simulink model "Nexonar_Test2"  (R2018b)
settings: Solver=FixedStepDiscrete  StartTime=0.0  StopTime=10  RelTol=1e-3  EnableMultiTasking=on
settings Model: ExtModeTrigDuration=8  Creator=User  LastModifiedBy=hengw
settings DataIOCC: LimitDataPoints=on  SaveFormat=Array  SaveOutput=off  SaveTime=off
settings OptimizationCC: DefaultUnderspecifiedDataType=single  ExpressionDepthLimit=2147483647  LifeSpan=1  MaxStackSize=512
settings DebuggingCC: UnderspecifiedInitializationDetection=Classic  MergeDetectMultiDrivingBlocksExec=none  SolverPrmCheckMsg=warning  StateNameClashWarn=warning  SFUnexpectedBacktrackingDiag=warning  SFNoUnconditionalDefaultTransitionDiag=warning  SFExecutionAtInitializationDiag=none
settings HardwareCC: ProdBitPerChar=16  ProdBitPerInt=16  ProdBitPerPointer=32  ProdBitPerSizeT=32  ProdBitPerPtrDiffT=32  ProdLargestAtomicInteger=Integer  ProdLargestAtomicFloat=None  ProdWordSize=16  ProdLongLongMode=on  ProdHWDeviceType=Texas Instruments->C2000  TargetBitPerChar=16  TargetBitPerInt=16  TargetLargestAtomicInteger=Integer  TargetIntDivRoundTo=Zero  TargetEndianess=LittleEndian  TargetWordSize=16  TargetHWDeviceType=Texas Instruments->C2000  ProdEqTarget=off
settings ModelReferenceCC: PropagateSignalLabelsOutOfModel=off
settings SFSimCC: SimCustomSourceCode="#include \"i2c_reset.c\""  SimCustomHeaderCode="#include \"i2c_reset.h\""  SimUseLocalCustomCode=off  MATLABDynamicMemAlloc=off
settings RTWCC: SystemTargetFile=ert.tlc  HardwareBoard=TI Delfino F2833x  TemplateMakefile=ert_default_tmf  RTWUseLocalCustomCode=off  RTWUseSimCustomCode=on  CustomSourceCode="#include \"i2c_reset.c\""  CustomHeaderCode="#include \"i2c_reset.h\""  Toolchain=Texas Instruments Code Composer Studio (C2000)
settings CodeAppCC: IgnoreCustomStorageClasses=off  CustomSymbolStrType=$N$R$M  StateflowObjectComments=on  InternalIdentifier=Classic
settings ERTTargetCC: CodeReplacementLibrary=TI C28x  MultiwordLength=2048  ParMdlRefBuildCompliant=off  CPPClassGenCompliant=off  ConvertIfToSwitch=off  SuppressUnreachableDefaultCases=off
settings ConfigComp: CovMetricSettings=dw  CovHtmlReporting=on  CovSaveCumulativeToWorkspaceVar=on  CovSaveSingleToWorkspaceVar=on  CovExternalEMLEnable=off

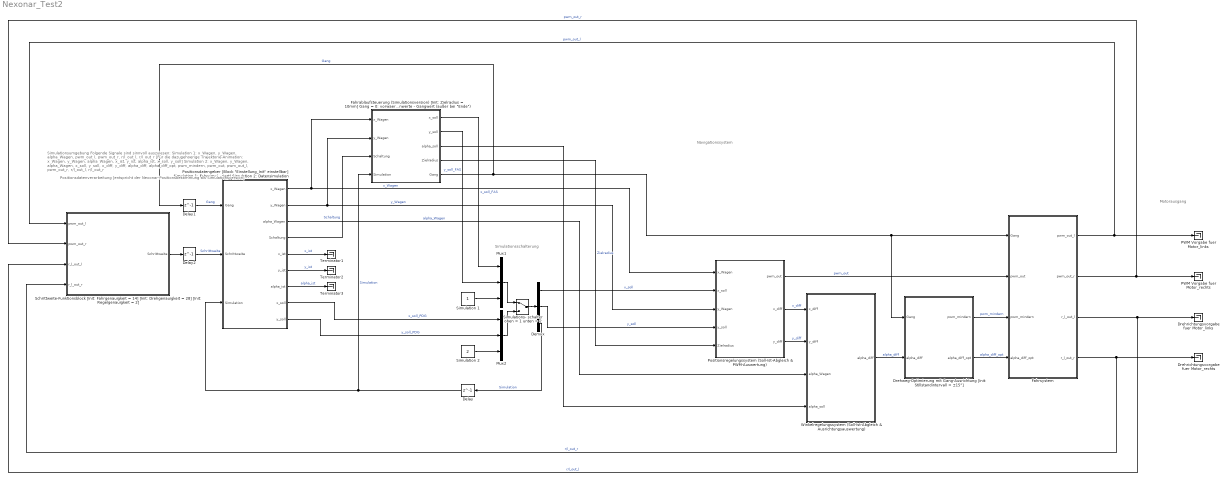
== system Nexonar_Test2 ==
  note: Simulationsschalterung
  note: Simulationsumgebung
      |
      |
      |
      |
      |
      |
      |
      |
      |
      |
      |
      |
      |
      |
      |
      |
      |
      |
      |
      |
      |
      |
      |
      |
      |
      |
      |
      |
      |
      |
      |
      |
      |
      |
      |
      |
      |
      |
      |
      |
      |
      | Folgende Signale sind sinnvoll auszulesen:
      | Simulation 1: x_Wagen, y_Wagen, alpha_Wagen, pwm_out_l, pwm_out_r, r/l_out_l, r/l_out_r
      | [Für die dazugehoerige Trajektorie-Animation: x_Wagen, y_Wagen, alpha_Wagen, x_ist, y_ist, alpha_ist, x_soll, y_soll]
      | Simulation 2: x_Wagen, y_Wagen, alpha_Wagen, x_soll, y_soll, x_diff, y_diff, alpha_diff, alpha_diff_opt, pwm_mindern, pwm_out, pwm_out_l, pwm_out_r, r/l_out_l, r/l_out_r
  note: Navigationssystem
  note: Motorausgang
  note: Positionsdatenverarbeitung
      |
      |
      |
      |
      |
      |
      |
      |
      |
      |
      |
      |
      |
      |
      |
      |
      |
      |
      |
      |
      |
      |
      |
      |
      |
      |
      |
      |
      |
      | [entspricht der Nexonar-Positionsbestimmung
      | als Simulationsversion]
  Delay : Delay  DelayLength=1  InitialCondition=0
  Delay1 : Delay  DelayLength=1  InitialCondition=0
  Delay2 : Delay  DelayLength=1  InitialCondition=0
  Demux : Demux  Outputs=3
  Drehrichtungsvorgabe fuer Motor_links : Terminator
  Drehrichtungsvorgabe fuer Motor_rechts : Terminator
  Drehweg-Optimierung mit Gang-Ausrichtung [Init: Stillstandintervall = ±15°] : Stateflow chart  TreatAsAtomicUnit=on
  "Fahrablaufsteuerung (Simulationsversion) [Init: Zielradius = 10mm] Gang = 0: vorwaerts Gang = 1: rueckwaerts Folgende Werte fuer den Ablauf sind einstellbar: - Zielkoordinatenwerte - Gangwert (außer bei \"Ende\")" : Stateflow chart  TreatAsAtomicUnit=on
  Fahrsystem : Stateflow chart  TreatAsAtomicUnit=on
  Mux1 : Mux  Inputs=3
  Mux2 : Mux  Inputs=3
  PWM Vorgabe fuer Motor_links : Terminator
  PWM Vorgabe fuer Motor_rechts : Terminator
  "Positionsdatengeber [Block \"Einstellung_Init\" einstellbar] Simulation 1: Fahrsimulation (Konvertierung integriert) Simulation 2: Datensimulation" : Stateflow chart  TreatAsAtomicUnit=on
  Positionsregelungssystem (Soll-Ist-Abgleich & PWM-Auswertung) : Subsystem
  Schrittweite-Funktionsblock [Init: Fahrgenauigkeit = 14] [Init: Drehgenauigkeit = 28] [Init: Regelgenauigkeit = 2] : MATLAB Function  TreatAsAtomicUnit=on
  Simulation 1 : Constant
  Simulation 2 : Constant  Value=2
  Simulations- schalter oben = 1 unten = 2 : ManualSwitch
  Terminator1 : Terminator
  Terminator2 : Terminator
  Terminator3 : Terminator
  Winkelregelungssystem (Soll-Ist-Abgleich & Ausrichtungsauswertung) : Subsystem
  wires:
  "Positionsdatengeber [Block \"Einstellung_Init\" einstellbar] Simulation 1: Fahrsimulation (Konvertierung integriert) Simulation 2: Datensimulation"/2(y_Wagen) -> Positionsregelungssystem (Soll-Ist-Abgleich & PWM-Auswertung)/3(y_Wagen), "Fahrablaufsteuerung (Simulationsversion) [Init: Zielradius = 10mm] Gang = 0: vorwaerts Gang = 1: rueckwaerts Folgende Werte fuer den Ablauf sind einstellbar: - Zielkoordinatenwerte - Gangwert (außer bei \"Ende\")"/2(y_Wagen)  "y_Wagen"
  Fahrsystem/4(r_l_out_r) -> Schrittweite-Funktionsblock [Init: Fahrgenauigkeit = 14] [Init: Drehgenauigkeit = 28] [Init: Regelgenauigkeit = 2]/4(r_l_out_r), Drehrichtungsvorgabe fuer Motor_rechts/1  "r/l_out_r"
  Fahrsystem/3(r_l_out_l) -> Drehrichtungsvorgabe fuer Motor_links/1, Schrittweite-Funktionsblock [Init: Fahrgenauigkeit = 14] [Init: Drehgenauigkeit = 28] [Init: Regelgenauigkeit = 2]/3(r_l_out_l)  "r/l_out_l"
  "Positionsdatengeber [Block \"Einstellung_Init\" einstellbar] Simulation 1: Fahrsimulation (Konvertierung integriert) Simulation 2: Datensimulation"/1(x_Wagen) -> Positionsregelungssystem (Soll-Ist-Abgleich & PWM-Auswertung)/1(x_Wagen), "Fahrablaufsteuerung (Simulationsversion) [Init: Zielradius = 10mm] Gang = 0: vorwaerts Gang = 1: rueckwaerts Folgende Werte fuer den Ablauf sind einstellbar: - Zielkoordinatenwerte - Gangwert (außer bei \"Ende\")"/1(x_Wagen)  "x_Wagen"
  Demux/1 -> Positionsregelungssystem (Soll-Ist-Abgleich & PWM-Auswertung)/2(x_soll)  "x_soll"
  Demux/2 -> Positionsregelungssystem (Soll-Ist-Abgleich & PWM-Auswertung)/4(y_soll)  "y_soll"
  Schrittweite-Funktionsblock [Init: Fahrgenauigkeit = 14] [Init: Drehgenauigkeit = 28] [Init: Regelgenauigkeit = 2]/1(Schrittweite) -> Delay2/1
  Fahrsystem/1(pwm_out_l) -> PWM Vorgabe fuer Motor_links/1, Schrittweite-Funktionsblock [Init: Fahrgenauigkeit = 14] [Init: Drehgenauigkeit = 28] [Init: Regelgenauigkeit = 2]/1(pwm_out_l)  "pwm_out_l"
  Fahrsystem/2(pwm_out_r) -> Schrittweite-Funktionsblock [Init: Fahrgenauigkeit = 14] [Init: Drehgenauigkeit = 28] [Init: Regelgenauigkeit = 2]/2(pwm_out_r), PWM Vorgabe fuer Motor_rechts/1  "pwm_out_r"
  Delay1/1 -> "Positionsdatengeber [Block \"Einstellung_Init\" einstellbar] Simulation 1: Fahrsimulation (Konvertierung integriert) Simulation 2: Datensimulation"/1(Gang)  "Gang"
  "Positionsdatengeber [Block \"Einstellung_Init\" einstellbar] Simulation 1: Fahrsimulation (Konvertierung integriert) Simulation 2: Datensimulation"/3(alpha_Wagen) -> Winkelregelungssystem (Soll-Ist-Abgleich & Ausrichtungsauswertung)/3(alpha_Wagen)  "alpha_Wagen"
  Simulation 1/1 -> Mux1/3
  Simulation 2/1 -> Mux2/3
  Demux/3 -> Delay/1  "Simulation"
  "Positionsdatengeber [Block \"Einstellung_Init\" einstellbar] Simulation 1: Fahrsimulation (Konvertierung integriert) Simulation 2: Datensimulation"/9(y_soll) -> Mux2/2  "y_soll_PDG"
  "Positionsdatengeber [Block \"Einstellung_Init\" einstellbar] Simulation 1: Fahrsimulation (Konvertierung integriert) Simulation 2: Datensimulation"/8(x_soll) -> Mux2/1  "x_soll_PDG"
  "Fahrablaufsteuerung (Simulationsversion) [Init: Zielradius = 10mm] Gang = 0: vorwaerts Gang = 1: rueckwaerts Folgende Werte fuer den Ablauf sind einstellbar: - Zielkoordinatenwerte - Gangwert (außer bei \"Ende\")"/2(y_soll) -> Mux1/2  "y_soll_FAS"
  "Fahrablaufsteuerung (Simulationsversion) [Init: Zielradius = 10mm] Gang = 0: vorwaerts Gang = 1: rueckwaerts Folgende Werte fuer den Ablauf sind einstellbar: - Zielkoordinatenwerte - Gangwert (außer bei \"Ende\")"/1(x_soll) -> Mux1/1  "x_soll_FAS"
  Delay2/1 -> "Positionsdatengeber [Block \"Einstellung_Init\" einstellbar] Simulation 1: Fahrsimulation (Konvertierung integriert) Simulation 2: Datensimulation"/2(Schrittweite)  "Schrittweite"
  "Positionsdatengeber [Block \"Einstellung_Init\" einstellbar] Simulation 1: Fahrsimulation (Konvertierung integriert) Simulation 2: Datensimulation"/4(Schaltung) -> "Fahrablaufsteuerung (Simulationsversion) [Init: Zielradius = 10mm] Gang = 0: vorwaerts Gang = 1: rueckwaerts Folgende Werte fuer den Ablauf sind einstellbar: - Zielkoordinatenwerte - Gangwert (außer bei \"Ende\")"/3(Schaltung)  "Schaltung"
  "Fahrablaufsteuerung (Simulationsversion) [Init: Zielradius = 10mm] Gang = 0: vorwaerts Gang = 1: rueckwaerts Folgende Werte fuer den Ablauf sind einstellbar: - Zielkoordinatenwerte - Gangwert (außer bei \"Ende\")"/4(Zielradius) -> Positionsregelungssystem (Soll-Ist-Abgleich & PWM-Auswertung)/5(Zielradius)  "Zielradius"
  Simulations- schalter oben = 1 unten = 2/1 -> Demux/1
  Mux2/1 -> Simulations- schalter oben = 1 unten = 2/2
  Mux1/1 -> Simulations- schalter oben = 1 unten = 2/1
  Delay/1 -> "Positionsdatengeber [Block \"Einstellung_Init\" einstellbar] Simulation 1: Fahrsimulation (Konvertierung integriert) Simulation 2: Datensimulation"/3(Simulation), "Fahrablaufsteuerung (Simulationsversion) [Init: Zielradius = 10mm] Gang = 0: vorwaerts Gang = 1: rueckwaerts Folgende Werte fuer den Ablauf sind einstellbar: - Zielkoordinatenwerte - Gangwert (außer bei \"Ende\")"/4(Simulation)  "Simulation"
  "Positionsdatengeber [Block \"Einstellung_Init\" einstellbar] Simulation 1: Fahrsimulation (Konvertierung integriert) Simulation 2: Datensimulation"/5(x_ist) -> Terminator1/1  "x_ist"
  "Positionsdatengeber [Block \"Einstellung_Init\" einstellbar] Simulation 1: Fahrsimulation (Konvertierung integriert) Simulation 2: Datensimulation"/6(y_ist) -> Terminator2/1  "y_ist"
  Drehweg-Optimierung mit Gang-Ausrichtung [Init: Stillstandintervall = ±15°]/2(alpha_diff_opt) -> Fahrsystem/4(alpha_diff_opt)  "alpha_diff_opt"
  Positionsregelungssystem (Soll-Ist-Abgleich & PWM-Auswertung)/3(y_diff) -> Winkelregelungssystem (Soll-Ist-Abgleich & Ausrichtungsauswertung)/2(y_diff)  "y_diff"
  Drehweg-Optimierung mit Gang-Ausrichtung [Init: Stillstandintervall = ±15°]/1(pwm_mindern) -> Fahrsystem/3(pwm_mindern)  "pwm_mindern"
  Winkelregelungssystem (Soll-Ist-Abgleich & Ausrichtungsauswertung)/1(alpha_diff) -> Drehweg-Optimierung mit Gang-Ausrichtung [Init: Stillstandintervall = ±15°]/2(alpha_diff)  "alpha_diff"
  Positionsregelungssystem (Soll-Ist-Abgleich & PWM-Auswertung)/2(x_diff) -> Winkelregelungssystem (Soll-Ist-Abgleich & Ausrichtungsauswertung)/1(x_diff)  "x_diff"
  "Fahrablaufsteuerung (Simulationsversion) [Init: Zielradius = 10mm] Gang = 0: vorwaerts Gang = 1: rueckwaerts Folgende Werte fuer den Ablauf sind einstellbar: - Zielkoordinatenwerte - Gangwert (außer bei \"Ende\")"/5(Gang) -> Fahrsystem/1(Gang), Drehweg-Optimierung mit Gang-Ausrichtung [Init: Stillstandintervall = ±15°]/1(Gang), Delay1/1  "Gang"
  Positionsregelungssystem (Soll-Ist-Abgleich & PWM-Auswertung)/1(pwm_out) -> Fahrsystem/2(pwm_out)  "pwm_out"
  "Positionsdatengeber [Block \"Einstellung_Init\" einstellbar] Simulation 1: Fahrsimulation (Konvertierung integriert) Simulation 2: Datensimulation"/7(alpha_ist) -> Terminator3/1  "alpha_ist"
  "Fahrablaufsteuerung (Simulationsversion) [Init: Zielradius = 10mm] Gang = 0: vorwaerts Gang = 1: rueckwaerts Folgende Werte fuer den Ablauf sind einstellbar: - Zielkoordinatenwerte - Gangwert (außer bei \"Ende\")"/3(alpha_soll) -> Winkelregelungssystem (Soll-Ist-Abgleich & Ausrichtungsauswertung)/4(alpha_soll)

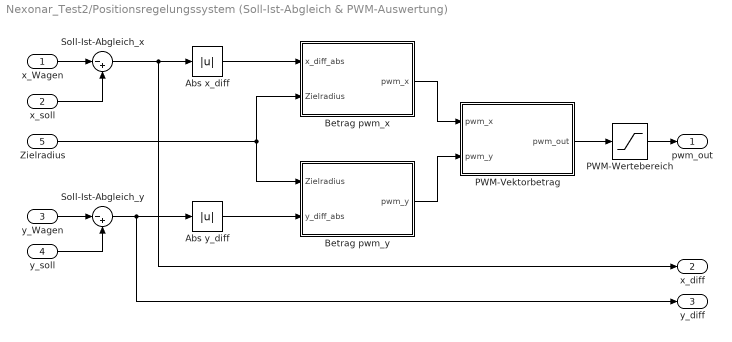
== system Nexonar_Test2/Positionsregelungssystem (Soll-Ist-Abgleich & PWM-Auswertung) ==
  x_Wagen : Inport
  x_soll : Inport  Port=2
  y_Wagen : Inport  Port=3
  y_soll : Inport  Port=4
  Zielradius : Inport  Port=5
  Abs x_diff : Abs  SampleTime=0.01
  Abs y_diff : Abs  SampleTime=0.01
  Betrag pwm_x : MATLAB Function  TreatAsAtomicUnit=on  SystemSampleTime=0.01
  Betrag pwm_y : MATLAB Function  TreatAsAtomicUnit=on  SystemSampleTime=0.01
  PWM-Vektorbetrag : MATLAB Function  TreatAsAtomicUnit=on
  PWM-Wertebereich : Saturate  UpperLimit=100  LowerLimit=0
  Soll-Ist-Abgleich_x : Sum  Inputs=|-+  SampleTime=0.01
  Soll-Ist-Abgleich_y : Sum  Inputs=|-+  AccumDataTypeStr=double  SampleTime=0.01
  pwm_out : Outport
  x_diff : Outport  Port=2
  y_diff : Outport  Port=3
  wires:
  Soll-Ist-Abgleich_x/1 -> x_diff/1, Abs x_diff/1
  Abs x_diff/1 -> Betrag pwm_x/1(x_diff_abs)
  x_soll/1 -> Soll-Ist-Abgleich_x/2
  x_Wagen/1 -> Soll-Ist-Abgleich_x/1
  y_Wagen/1 -> Soll-Ist-Abgleich_y/1
  y_soll/1 -> Soll-Ist-Abgleich_y/2
  Soll-Ist-Abgleich_y/1 -> Abs y_diff/1, y_diff/1
  Abs y_diff/1 -> Betrag pwm_y/2(y_diff_abs)
  PWM-Wertebereich/1 -> pwm_out/1
  PWM-Vektorbetrag/1(pwm_out) -> PWM-Wertebereich/1
  Betrag pwm_x/1(pwm_x) -> PWM-Vektorbetrag/1(pwm_x)
  Betrag pwm_y/1(pwm_y) -> PWM-Vektorbetrag/2(pwm_y)
  Zielradius/1 -> Betrag pwm_y/1(Zielradius), Betrag pwm_x/2(Zielradius)

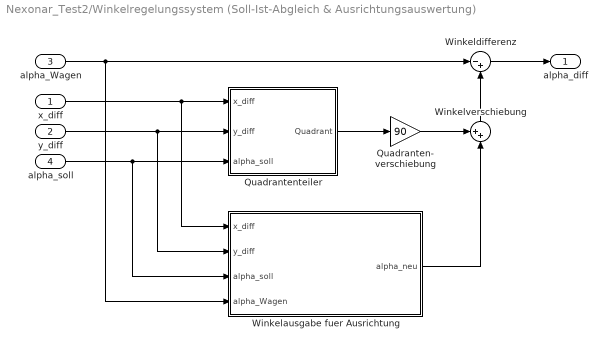
== system Nexonar_Test2/Winkelregelungssystem (Soll-Ist-Abgleich & Ausrichtungsauswertung) ==
  x_diff : Inport
  y_diff : Inport  Port=2
  alpha_Wagen : Inport  Port=3
  alpha_soll : Inport  Port=4
  Quadranten- verschiebung : Gain  Gain=90
  Quadrantenteiler : Stateflow chart  TreatAsAtomicUnit=on
  Winkelausgabe fuer Ausrichtung : Stateflow chart  TreatAsAtomicUnit=on
  Winkeldifferenz : Sum  Inputs=|-+
  Winkelverschiebung : Sum  Inputs=++|
  alpha_diff : Outport
  wires:
  alpha_Wagen/1 -> Winkelausgabe fuer Ausrichtung/4(alpha_Wagen), Winkeldifferenz/1
  y_diff/1 -> Winkelausgabe fuer Ausrichtung/2(y_diff), Quadrantenteiler/2(y_diff)
  Winkelausgabe fuer Ausrichtung/1(alpha_neu) -> Winkelverschiebung/2
  Winkelverschiebung/1 -> Winkeldifferenz/2
  x_diff/1 -> Winkelausgabe fuer Ausrichtung/1(x_diff), Quadrantenteiler/1(x_diff)
  Quadrantenteiler/1(Quadrant) -> Quadranten- verschiebung/1
  Winkeldifferenz/1 -> alpha_diff/1
  Quadranten- verschiebung/1 -> Winkelverschiebung/1
  alpha_soll/1 -> Winkelausgabe fuer Ausrichtung/3(alpha_soll), Quadrantenteiler/3(alpha_soll)

== stateflow chart Nexonar_Test2/Fahrablaufsteuerung (Simulationsversion) [Init: Zielradius = 10mm] Gang = 0: vorwaerts Gang = 1: rueckwaerts Folgende Werte fuer den Ablauf sind einstellbar: - Zielkoordinatenwerte - Gangwert (außer bei "Ende") ==
  state Start_Einstellung_Init
    entry:
    Zielradius = 10;
  state Sammeln1 [commented out]
    state Anfahrpunkt_1 [commented out]
      entry:
      x_soll = 1500;
      y_soll = 0;
      alpha_soll = -1;
    state Wechsel_1 [commented out]
      entry:
      Counter = Counter + 1;
    state Anfahrpunkt_2 [commented out]
      entry:
      x_soll = 1200;
      y_soll = 100;
      alpha_soll = -1;
    state Wechsel_2 [commented out]
      entry:
      Counter = Counter + 1;
    state Anfahrpunkt_3 [commented out]
      entry:
      x_soll = 1000;
      y_soll = 250;
      alpha_soll = -1;
    state Wechsel_3 [commented out]
      entry:
      Counter = Counter + 1;
    state Anfahrpunkt_4 [commented out]
      entry:
      x_soll = 940;
      y_soll = 650;
      alpha_soll = -1;
    state Wechsel_4 [commented out]
      entry:
      Counter = Counter + 1;
    state Anfahrpunkt_5 [commented out]
      entry:
      x_soll = 850;
      y_soll = 750;
      alpha_soll = -1;
    state Wechsel_5 [commented out]
      entry:
      Counter = Counter + 1;
    state Anfahrpunkt_6 [commented out]
      entry:
      x_soll = 600;
      y_soll = 825;
      alpha_soll = -1;
    state Wechsel_6 [commented out]
      entry:
      Counter = Counter + 1;
    state Wechsel_10 [commented out]
      entry:
      Counter = Counter + 1;
    state Anfahrpunkt_7 [commented out]
      entry:
      x_soll = 500;
      y_soll = 825;
      alpha_soll = -1;
    state Anfahrpunkt_10 [commented out]
      entry:
      x_soll = 880;
      y_soll = 0;
      alpha_soll = -1;
    state Wechsel_7 [commented out]
      entry:
      Counter = Counter + 1;
    state Anfahrpunkt_8 [commented out]
      entry:
      x_soll = 325;
      y_soll = 725;
      alpha_soll = -1;
    state Wechsel_8 [commented out]
      entry:
      Counter = Counter + 1;
    state Anfahrpunkt_9 [commented out]
      entry:
      x_soll = 400;
      y_soll = 300;
      alpha_soll = -1;
    state Wechsel_9 [commented out]
      entry:
      Counter = Counter + 1;
    state Anfahrpunkt_11 [commented out]
      entry:
      x_soll = 600;
      y_soll = 0;
      alpha_soll = -1;
    state Wechsel_11 [commented out]
      entry:
      Counter = Counter + 1;
    state Anfahrpunkt_12 [commented out]
      entry:
      x_soll = 900;
      y_soll = 0;
      alpha_soll = -1;
    state Wechsel_12 [commented out]
      entry:
      Counter = Counter + 1;
    state Anfahrpunkt_13 [commented out]
      entry:
      x_soll = 1200;
      y_soll = 0;
      alpha_soll = -1;
    state Wechsel_13 [commented out]
      entry:
      Counter = Counter + 1;
    state Anfahrpunkt_14 [commented out]
      entry:
      x_soll = 1420;
      y_soll = -100;
      alpha_soll = -1;
    state Wechsel_14 [commented out]
      entry:
      Counter = Counter + 1;
    (default) -> Anfahrpunkt_1 [commented out] : {Counter = 0}
    Anfahrpunkt_1 -> Sammeln1.Wechsel_1 [commented out] : [abs(x_soll - x_Wagen) <= Zielradius && abs(y_soll - y_Wagen) <= Zielradius]
    Sammeln1.Wechsel_1 -> Anfahrpunkt_2 [commented out]
    Anfahrpunkt_2 -> Sammeln1.Wechsel_2 [commented out] : [abs(x_soll - x_Wagen) <= Zielradius && abs(y_soll - y_Wagen) <= Zielradius]
    Sammeln1.Wechsel_2 -> Anfahrpunkt_3 [commented out]
    Anfahrpunkt_3 -> Sammeln1.Wechsel_3 [commented out] : [abs(x_soll - x_Wagen) <= Zielradius && abs(y_soll - y_Wagen) <= Zielradius]
    Sammeln1.Wechsel_3 -> Anfahrpunkt_4 [commented out]
    Wechsel_10 -> Anfahrpunkt_4 [commented out]
    Anfahrpunkt_4 -> Wechsel_4 [commented out] : [abs(x_soll - x_Wagen) <= Zielradius && abs(y_soll - y_Wagen) <= Zielradius]
    Wechsel_4 -> Anfahrpunkt_5 [commented out]
    Anfahrpunkt_5 -> Wechsel_5 [commented out] : [abs(x_soll - x_Wagen) <= Zielradius && abs(y_soll - y_Wagen) <= Zielradius]
    Wechsel_5 -> Anfahrpunkt_6 [commented out]
    Anfahrpunkt_6 -> Wechsel_6 [commented out] : [abs(x_soll - x_Wagen) <= Zielradius && abs(y_soll - y_Wagen) <= Zielradius]
    Wechsel_6 -> Anfahrpunkt_7 [commented out]
    Anfahrpunkt_10 -> Wechsel_10 [commented out] : [abs(x_soll - x_Wagen) <= Zielradius && abs(y_soll - y_Wagen) <= Zielradius]
    Anfahrpunkt_7 -> Wechsel_7 [commented out] : [abs(x_soll - x_Wagen) <= Zielradius && abs(y_soll - y_Wagen) <= Zielradius]
    Wechsel_9 -> Anfahrpunkt_10 [commented out] : [Counter == 9]
    Wechsel_7 -> Anfahrpunkt_8 [commented out]
    Anfahrpunkt_8 -> Wechsel_8 [commented out] : [abs(x_soll - x_Wagen) <= Zielradius && abs(y_soll - y_Wagen) <= Zielradius]
    Wechsel_8 -> Anfahrpunkt_9 [commented out]
    Anfahrpunkt_9 -> Wechsel_9 [commented out] : [abs(x_soll - x_Wagen) <= Zielradius && abs(y_soll - y_Wagen) <= Zielradius]
    Wechsel_9 -> Anfahrpunkt_11 [commented out]
    Anfahrpunkt_11 -> Wechsel_11 [commented out] : [abs(x_soll - x_Wagen) <= Zielradius && abs(y_soll - y_Wagen) <= Zielradius]
    Wechsel_11 -> Anfahrpunkt_12 [commented out]
    Anfahrpunkt_12 -> Wechsel_12 [commented out] : [abs(x_soll - x_Wagen) <= Zielradius && abs(y_soll - y_Wagen) <= Zielradius]
    Wechsel_12 -> Anfahrpunkt_13 [commented out]
    Anfahrpunkt_13 -> Wechsel_13 [commented out] : [abs(x_soll - x_Wagen) <= Zielradius && abs(y_soll - y_Wagen) <= Zielradius]
    Wechsel_13 -> Sammeln1.Anfahrpunkt_14 [commented out]
    Sammeln1.Anfahrpunkt_14 -> Sammeln1.Wechsel_14 [commented out] : [abs(x_soll - x_Wagen) <= Zielradius && abs(y_soll - y_Wagen) <= Zielradius]
  state Parken
    state Parken_1
      entry:
      x_soll = 1420;
      y_soll = -50;
      alpha_soll = -1;
    state Wechsel_1
      entry:
      Counter = Counter + 1;
    state Parken_2
      entry:
      x_soll = 1620;
      y_soll = -135;
      alpha_soll = -1;
    state Wechsel_2
      entry:
      Counter = Counter + 1;
    state Parken_3
      entry:
      x_soll = 1640;
      y_soll = -131;
      alpha_soll = -1;
    state Wechsel_3
      entry:
      Counter = Counter + 1;
    (default) -> Parken_1 : {Counter = 0}
    Parken_1 -> Parken.Wechsel_1 : [abs(x_soll - x_Wagen) <= Zielradius && abs(y_soll - y_Wagen) <= Zielradius]
    Parken.Wechsel_1 -> Parken_2
    Parken_2 -> Parken.Wechsel_2 : [abs(x_soll - x_Wagen) <= Zielradius && abs(y_soll - y_Wagen) <= Zielradius]
    Parken.Wechsel_2 -> Parken_3
    Parken_3 -> Parken.Wechsel_3 : [abs(x_soll - x_Wagen) <= Zielradius && abs(y_soll - y_Wagen) <= Zielradius]
  state Uebergabe
    state Uebergabepunkt_x_Richtung
      entry:
      x_soll = x_least;
      y_soll = y_least;
      alpha_soll = -1;
    state Wechsel_1
      entry:
      Counter = Counter + 1;
    state Uebergabepunkt_y_Richtung
      entry:
      x_soll = x_least;
      y_soll = 5;
      alpha_soll = 90;
    state Warten_Uebergabe
    state Wechsel_2
      entry:
      Counter = Counter + 1;
    (default) -> Uebergabepunkt_x_Richtung : {Counter = 0}
    Uebergabepunkt_x_Richtung -> Uebergabe.Wechsel_1 : [abs(x_soll - x_Wagen) <= Zielradius && abs(y_soll - y_Wagen) <= Zielradius]
        | {x_least = x_soll; y_least = y_soll;}
    Uebergabe.Wechsel_1 -> Uebergabepunkt_y_Richtung
    Uebergabepunkt_y_Richtung -> Warten_Uebergabe : [abs(x_soll - x_Wagen) <= Zielradius && abs(y_soll - y_Wagen) <= Zielradius]
    Warten_Uebergabe -> Uebergabe.Wechsel_2 : [after(1,sec)]
  state Sammeln
    state Anfahrpunkt_14
      entry:
      x_soll = 1420;
      y_soll = -100;
      alpha_soll = -1;
    state Wechsel_14
      entry:
      Counter = Counter + 1;
    (default) -> Sammeln.Anfahrpunkt_14 : {Counter = 0}
    Sammeln.Anfahrpunkt_14 -> Sammeln.Wechsel_14 : [abs(x_soll - x_Wagen) <= Zielradius && abs(y_soll - y_Wagen) <= Zielradius]
  state Schaltung_Gang_Weiterleitung
    Gang = Schaltung;
  state Ende
    entry:
    Gang = 2;
  (default) -> Start_Einstellung_Init
  Sammeln1 -> ? [commented out] : [Counter == 20]
      | {Gang = 1;
      | x_least = x_soll;
      | y_least = y_soll;}
  Start_Einstellung_Init -> (junction 137)
  (junction 137) -> Schaltung_Gang_Weiterleitung [order 2]
  (junction 137) -> Sammeln [order 1] : [Simulation == 1]{Gang = 0}
  Uebergabe -> Parken : [Counter == 2]{Gang = 0}
  Sammeln -> Uebergabe : [Counter == 1]
      | {Gang = 1;
      | x_least = x_soll;
      | y_least = y_soll;}
  Parken -> Ende : [Counter == 3]
  data: x_soll output; y_soll output; alpha_soll output; Zielradius output; x_Wagen input; y_Wagen input; Counter local; x_least local; y_least local; Schaltung input; Simulation input; Gang output

== matlab function Nexonar_Test2/Positionsregelungssystem (Soll-Ist-Abgleich & PWM-Auswertung)/PWM-Vektorbetrag ==
  data: pwm_x input; pwm_out output; pwm_y input
function pwm_out = fcn(pwm_x, pwm_y)

pwm_out = round(sqrt(pwm_x * pwm_x + pwm_y * pwm_y));

== stateflow chart Nexonar_Test2/Positionsdatengeber [Block "Einstellung_Init" einstellbar] Simulation 1: Fahrsimulation (Konvertierung integriert) Simulation 2: Datensimulation ==
  state Start_Init_Fahrsimulation
    alpha_ist = Start_alpha;
    x_ist = Start_x;
    y_ist = Start_y;
    alpha_Wagen = alpha_ist - psi_Offset_Nexo;
    x_Wagen = x_ist - round(r_Versatz_Nexo * cos((phi_Versatz_Nexo+alpha_Wagen)*2*pi/360));
    y_Wagen = y_ist - round(r_Versatz_Nexo * sin((phi_Versatz_Nexo+alpha_Wagen)*2*pi/360));;
    x_soll = 0;
    y_soll = 0;
  state Fahrsimulation
    state Fahren_mit_Ausrichtungsregelung
      alpha_ist = alpha_ist + Schrittweite(2);
      alpha_Wagen = alpha_Wagen + Schrittweite(2);
      x_ist = x_ist + round(Schrittweite(1) * cos(alpha_Wagen*2*pi/360+pi*Schaltung));
      y_ist = y_ist + round(Schrittweite(1) * sin(alpha_Wagen*2*pi/360+pi*Schaltung));
      x_Wagen = x_ist - round(r_Versatz_Nexo * cos((phi_Versatz_Nexo+alpha_Wagen)*2*pi/360));
      y_Wagen = y_ist - round(r_Versatz_Nexo * sin((phi_Versatz_Nexo+alpha_Wagen)*2*pi/360));
    state Drehen
      alpha_ist = alpha_ist + Schrittweite(2);
      alpha_Wagen = alpha_Wagen + Schrittweite(2);
      x_ist = x_Wagen + round(r_Versatz_Nexo * cos((phi_Versatz_Nexo+alpha_Wagen)*2*pi/360));
      y_ist = y_Wagen + round(r_Versatz_Nexo * sin((phi_Versatz_Nexo+alpha_Wagen)*2*pi/360));
    (junction 192) -> (junction 250) [order 1] : [alpha_Wagen + Schrittweite(2) >= 360]
        | {alpha_Wagen = alpha_Wagen - 360}
    (junction 190) -> (junction 192) [order 1] : [alpha_ist + Schrittweite(2) >= 360]
        | {alpha_ist = alpha_ist - 360}
    (junction 250) -> Fahren_mit_Ausrichtungsregelung [order 2]
    Fahren_mit_Ausrichtungsregelung -> (junction 138)
    (junction 192) -> (junction 250) [order 2] : [alpha_Wagen + Schrittweite(2) < 0]
        | {alpha_Wagen = alpha_Wagen + 360}
    (junction 190) -> (junction 192) [order 2] : [alpha_ist + Schrittweite(2) < 0]
        | {alpha_ist = alpha_ist + 360}
    Drehen -> (junction 138)
    (default) -> (junction 190)
    (junction 190) -> (junction 192) [order 3]
    (junction 192) -> (junction 250) [order 3]
    (junction 250) -> Drehen [order 1] : [Schrittweite(1) == 0]
    (junction 138) -> (junction 190) : {Schaltung = Gang}
  state Einstellung_Init
    %% Einstellungen allgemein
    Start_x = 900;
    Start_y = 0;
    Start_alpha = 15 % nur 0 – 359 in Fahrsimulation
    %% Einstellungen für Fahrsimulation
    r_Versatz_Nexo = 2.5;
    phi_Versatz_Nexo = 30;
    psi_Offset_Nexo = 15;
    %% Einstellungen für Datensimulation
    Anfang_x = 0;
    Anfang_y = 0;
    Pos_max = 1000;
    Winkel_max = 360;
    Pos_Schritt = 200;   % > 0
    Winkel_Schritt = 20; % > 0
  state Ende
  state Start_Init_Datensimulation
    alpha_ist = 0;
    x_ist = 0;
    y_ist = 0;
    alpha_Wagen = Start_alpha;
    x_Wagen = Start_x;
    y_Wagen = Start_y;
    x_soll = Anfang_x;
    y_soll = Anfang_y;
  state Datensimulation
    state x_Wagen_Counter
      x_Wagen = x_Wagen + Pos_Schritt;
    state y_Wagen_Counter
      y_Wagen = y_Wagen + Pos_Schritt;
    state x_soll_Counter
      x_soll = x_soll + Pos_Schritt;
    state y_soll_Counter
      y_soll = y_soll + Pos_Schritt;
    state alpha_Wagen_Counter
      alpha_Wagen = alpha_Wagen + Winkel_Schritt;
    state Gangwechsel
      Schaltung = Schaltung + 1;
    (junction 195) -> Gangwechsel [order 2] : [y_Wagen + Pos_Schritt > Pos_max && x_soll + Pos_Schritt > Pos_max && y_soll + Pos_Schritt > Pos_max && alpha_Wagen + Winkel_Schritt >= Winkel_max]
        | {x_Wagen = Start_x; y_Wagen = Start_y; x_soll = Anfang_x; y_soll = Anfang_y, alpha_Wagen = Start_alpha;}
    (junction 195) -> alpha_Wagen_Counter [order 3] : [y_Wagen + Pos_Schritt > Pos_max && x_soll + Pos_Schritt > Pos_max && y_soll + Pos_Schritt > Pos_max]
        | {x_Wagen = Start_x; y_Wagen = Start_y; x_soll = Anfang_x; y_soll = Anfang_y;}
    (default) -> (junction 195)
    (junction 195) -> y_soll_Counter [order 4] : [y_Wagen + Pos_Schritt > Pos_max && x_soll + Pos_Schritt > Pos_max]
        | {x_Wagen = Start_x; y_Wagen = Start_y;
        | x_soll = Anfang_x;}
    (junction 195) -> x_soll_Counter [order 5] : [y_Wagen + Pos_Schritt > Pos_max]
        | {x_Wagen = Start_x;
        | y_Wagen = Start_y;}
    Gangwechsel -> (junction 195)
    alpha_Wagen_Counter -> (junction 195)
    y_soll_Counter -> (junction 195)
    x_soll_Counter -> (junction 195)
    (junction 195) -> y_Wagen_Counter [order 6] : {x_Wagen = Start_x}
    y_Wagen_Counter -> (junction 195)
    (junction 195) -> x_Wagen_Counter [order 1] : [x_Wagen + Pos_Schritt <= Pos_max]
    x_Wagen_Counter -> (junction 195)
  (junction 102) -> Start_Init_Fahrsimulation [order 1] : [Simulation == 1]
  Fahrsimulation -> Ende : [Schaltung == 2]
  Start_Init_Fahrsimulation -> Fahrsimulation : {Schaltung = Gang}
  Einstellung_Init -> (junction 102)
  (default) -> Einstellung_Init
  (junction 102) -> Start_Init_Datensimulation [order 2]
  Datensimulation -> Ende : [Schaltung == 2]
  Start_Init_Datensimulation -> Datensimulation : {Schaltung = 0}
  data: x_Wagen output; y_Wagen output; alpha_Wagen output; Schaltung output; Gang input double; x_ist output; y_ist output; alpha_ist output; Pos_max local; Pos_Schritt local; Winkel_Schritt local; Schrittweite input double; Simulation input; Start_x local; Start_y local; Start_alpha local; Anfang_x local; Anfang_y local; Winkel_max local; r_Versatz_Nexo local; phi_Versatz_Nexo local; x_soll output; y_soll output; psi_Offset_Nexo local

== matlab function Nexonar_Test2/Schrittweite-Funktionsblock [Init: Fahrgenauigkeit = 14] [Init: Drehgenauigkeit = 28] [Init: Regelgenauigkeit = 2] ==
  data: pwm_out_l input; Schrittweite output; pwm_out_r input; r_l_out_l input; r_l_out_r input
function Schrittweite = fcn(pwm_out_l, pwm_out_r, r_l_out_l, r_l_out_r)

Fahrgenauigkeit = 14; % bis 141
Drehgenauigkeit = 28; % bis 141
Regelgenauigkeit = 1; % bis 10


Schrittweite = [0 0];
if r_l_out_l == r_l_out_r
    Schrittweite(1) = round(sqrt(pwm_out_l * pwm_out_l + pwm_out_r * pwm_out_r) / Fahrgenauigkeit);
    % Fahren Wertebereich brutto: 0 - 141
    Schrittweite(2) = round((pwm_out_r - pwm_out_l) / Regelgenauigkeit) * (1 + (r_l_out_l - 1) * 2);
    % Fahrregelung Wertebereich brutto: 0 - 10
else
    Schrittweite(1) = 0;
    Schrittweite(2) = round(sqrt(pwm_out_l * pwm_out_l + pwm_out_r * pwm_out_r) / Drehgenauigkeit) * (r_l_out_r - r_l_out_l);
    % Drehen Wertebereich brutto: 0 - 141
end

== stateflow chart Nexonar_Test2/Fahrsystem ==
  state Fahren_mit_Ausrichtungsregelung
    entry:
    pwm_out_l = pwm_out - round(pwm_mindern(1) * (pwm_out / 100) ^ 2) * l_mindern;
    pwm_out_r = pwm_out - round(pwm_mindern(1) * (pwm_out / 100) ^ 2) * r_mindern;
    r_l_out_l = 1 - Gang;
    r_l_out_r = 1 - Gang;
  state Start_Warten
  state Drehen_links_max
    entry:
    pwm_out_l = 100;
    pwm_out_r = 100;
    r_l_out_l = 0;
    r_l_out_r = 1;
  state Drehen_rechts_max
    entry:
    pwm_out_l = 100;
    pwm_out_r = 100;
    r_l_out_l = 1;
    r_l_out_r = 0;
  state Drehen_links_gesteuert
    entry:
    pwm_out_l = 59 + abs(alpha_diff_opt);
    pwm_out_r = 59 + abs(alpha_diff_opt);
    r_l_out_l = 0;
    r_l_out_r = 1;
  state Drehen_rechts_gesteuert
    entry:
    pwm_out_l = 59 + abs(alpha_diff_opt);
    pwm_out_r = 59 + abs(alpha_diff_opt);
    r_l_out_l = 1;
    r_l_out_r = 0;
  (junction 81) -> Fahren_mit_Ausrichtungsregelung [order 1] : [pwm_mindern(2) == 1]
      | {l_mindern = 1 - Gang; r_mindern = 0 + Gang;}
  (junction 81) -> Fahren_mit_Ausrichtungsregelung [order 2] : [pwm_mindern(2) == 0]
      | {l_mindern = 0 + Gang; r_mindern = 1 - Gang;}
  (junction 1) -> (junction 81) [order 2]
  Fahren_mit_Ausrichtungsregelung -> (junction 32)
  (junction 81) -> Fahren_mit_Ausrichtungsregelung [order 3] : {l_mindern = 0; r_mindern = 0;}
  Start_Warten -> (junction 1)
  (junction 32) -> (junction 1)
  (default) -> Start_Warten
  Drehen_links_max -> (junction 32)
  Drehen_rechts_max -> (junction 32)
  Drehen_links_gesteuert -> (junction 32)
  (junction 1) -> (junction 18) [order 1] : [abs(alpha_diff_opt) > 0 && pwm_out > 0]
  Drehen_rechts_gesteuert -> (junction 32)
  (junction 18) -> (junction 44) [order 1] : [abs(alpha_diff_opt) > 40]
  (junction 44) -> Drehen_links_max [order 1] : [alpha_diff_opt > 0]
  (junction 18) -> (junction 52) [order 2]
  (junction 44) -> Drehen_rechts_max [order 2]
  (junction 52) -> Drehen_links_gesteuert [order 1] : [alpha_diff_opt > 0]
  (junction 52) -> Drehen_rechts_gesteuert [order 2]
  data: Gang input; pwm_out input; pwm_mindern input; alpha_diff_opt input; pwm_out_l output; pwm_out_r output; r_l_out_l output; r_l_out_r output; l_mindern local; r_mindern local

== stateflow chart Nexonar_Test2/Drehweg-Optimierung mit Gang-Ausrichtung [Init: Stillstandintervall = ±15°] ==
  state Einstellung_Init
    entry:
    Stillstandintervall = 15;
    %%%
    pwm_mindern = [0 0];
  state Drehstillstand_mit_Ausrichtungsregelung
    entry:
    alpha_diff_opt = 0;
    if abs(alpha_diff_intern) < 5
    pwm_mindern(1) = round(abs(alpha_diff_intern));
    elseif abs(alpha_diff_intern) < 15
    pwm_mindern(1) = 5 + floor((abs(alpha_diff_intern) - 5) / 2);
    else
    pwm_mindern(1) = 10;
    end;
    if alpha_diff_intern < 0
    pwm_mindern(2) = 0;
    elseif alpha_diff_intern > 0
    pwm_mindern(2) = 1;
    else
    pwm_mindern(2) = 2;
    end;
  state Weiterleitung_bei_Drehzustand
    entry:
    alpha_diff_opt = alpha_diff_intern;
  (default) -> Einstellung_Init
  (junction 95) -> (junction 32)
  Einstellung_Init -> (junction 32)
  (junction 32) -> (junction 6) : {alpha_diff_intern = alpha_diff + 180 * Gang}
  (junction 6) -> (junction 68) [order 2]
  (junction 68) -> Drehstillstand_mit_Ausrichtungsregelung [order 1] : [abs(alpha_diff_intern) <= Stillstandintervall]
  Drehstillstand_mit_Ausrichtungsregelung -> (junction 95)
  (junction 6) -> (junction 13) [order 1] : [abs(alpha_diff_intern) > 180]
  (junction 13) -> (junction 68) [order 1] : [alpha_diff_intern > 0]
      | {alpha_diff_intern = -360 + alpha_diff_intern}
  Weiterleitung_bei_Drehzustand -> (junction 95)
  (junction 13) -> (junction 68) [order 2] : {alpha_diff_intern = 360 + alpha_diff_intern}
  (junction 68) -> Weiterleitung_bei_Drehzustand [order 2]
  data: pwm_mindern output; Gang input; alpha_diff input; alpha_diff_opt output; alpha_diff_intern local; Stillstandintervall local

== stateflow chart Nexonar_Test2/Winkelregelungssystem (Soll-Ist-Abgleich & Ausrichtungsauswertung)/Quadrantenteiler ==
  state Quadrant_a
    entry:
    Quadrant = 0;
  state Quadrant_b
    entry:
    Quadrant = 1;
  state Start_Warten
  state Quadrant_c
    entry:
    Quadrant = 2;
  state Quadrant_d
    entry:
    Quadrant = 3;
  (junction 6) -> Quadrant_a [order 1] : [alpha_soll ~= -1]
  Quadrant_a -> (junction 35)
  (junction 6) -> Quadrant_a [order 2] : [x_diff >= 0 && y_diff >= 0]
  (junction 6) -> Quadrant_b [order 3] : [x_diff <= 0 && y_diff > 0]
  Quadrant_b -> (junction 35)
  Start_Warten -> (junction 6)
  (junction 35) -> (junction 6)
  (default) -> Start_Warten
  (junction 6) -> Quadrant_c [order 4] : [x_diff < 0 && y_diff <= 0]
  Quadrant_c -> (junction 35)
  (junction 6) -> Quadrant_d [order 5]
  Quadrant_d -> (junction 35)
  data: x_diff input; y_diff input; Quadrant output; alpha_soll input

== stateflow chart Nexonar_Test2/Winkelregelungssystem (Soll-Ist-Abgleich & Ausrichtungsauswertung)/Winkelausgabe fuer Ausrichtung ==
  state Ausrichtung_gegeben
    entry:
    alpha_neu = alpha_soll;
  state Ausrichtung_ohne_Aenderung
    entry:
    alpha_neu = alpha_Wagen;
  state Start_Warten
  state Trigonometrische_Auswertung_in_Grad_fuer_Quadrant_1_3
    entry:
    alpha_neu = round(atan(abs(x_diff)/abs(y_diff))*360/(2*pi));
  state Trigonometrische_Auswertung_in_Grad_fuer_Quadrant_0_2
    entry:
    alpha_neu = round(atan(abs(y_diff)/abs(x_diff))*360/(2*pi));
  Ausrichtung_gegeben -> (junction 65)
  (junction 4) -> Ausrichtung_gegeben [order 1] : [alpha_soll ~= -1]
  (junction 4) -> Ausrichtung_ohne_Aenderung [order 2] : [x_diff == 0 && y_diff == 0]
  Ausrichtung_ohne_Aenderung -> (junction 65)
  Start_Warten -> (junction 4)
  (junction 65) -> (junction 4)
  (default) -> Start_Warten
  (junction 4) -> Trigonometrische_Auswertung_in_Grad_fuer_Quadrant_1_3 [order 5]
  Trigonometrische_Auswertung_in_Grad_fuer_Quadrant_1_3 -> (junction 65)
  (junction 4) -> Trigonometrische_Auswertung_in_Grad_fuer_Quadrant_0_2 [order 3] : [x_diff > 0 && y_diff >= 0]
  (junction 4) -> Trigonometrische_Auswertung_in_Grad_fuer_Quadrant_0_2 [order 4] : [x_diff < 0 && y_diff <= 0]
  Trigonometrische_Auswertung_in_Grad_fuer_Quadrant_0_2 -> (junction 65)
  data: x_diff input; y_diff input; alpha_soll input; alpha_neu output; alpha_Wagen input

== matlab function Nexonar_Test2/Positionsregelungssystem (Soll-Ist-Abgleich & PWM-Auswertung)/Betrag pwm_x ==
  settings: updateMethod=DISCRETE  sampleTime=0.01
  data: x_diff_abs input; pwm_x output; Zielradius input
function pwm_x = fcn( x_diff_abs, Zielradius)

if Zielradius < x_diff_abs && x_diff_abs < 60 + Zielradius
    pwm_x = 60;
elseif x_diff_abs <= Zielradius
    pwm_x = 0;
elseif x_diff_abs >= 100 + Zielradius
    pwm_x = 100;
else
    pwm_x = x_diff_abs;
end

== matlab function Nexonar_Test2/Positionsregelungssystem (Soll-Ist-Abgleich & PWM-Auswertung)/Betrag pwm_y ==
  settings: updateMethod=DISCRETE  sampleTime=0.01
  data: Zielradius input; y_diff_abs input; pwm_y output
function pwm_y = fcn(Zielradius, y_diff_abs)

if Zielradius < y_diff_abs && y_diff_abs < 60 + Zielradius
    pwm_y = 60;
elseif y_diff_abs <= Zielradius
    pwm_y = 0;
elseif y_diff_abs >= 100 + Zielradius
    pwm_y = 100;
else
    pwm_y = y_diff_abs;
end
